simulink model "detumbling"  (R2020b)
settings: Solver=ode15s  StartTime=0  StopTime=900  MaxStep=0.1  RelTol=1e-8  AbsTol=1e-8
values from neighbouring files (symbols this model uses):
  data = struct()    [config.m]
libraries: simulink x3
settings Model: Creator=pacif  LastModifiedBy=pacif

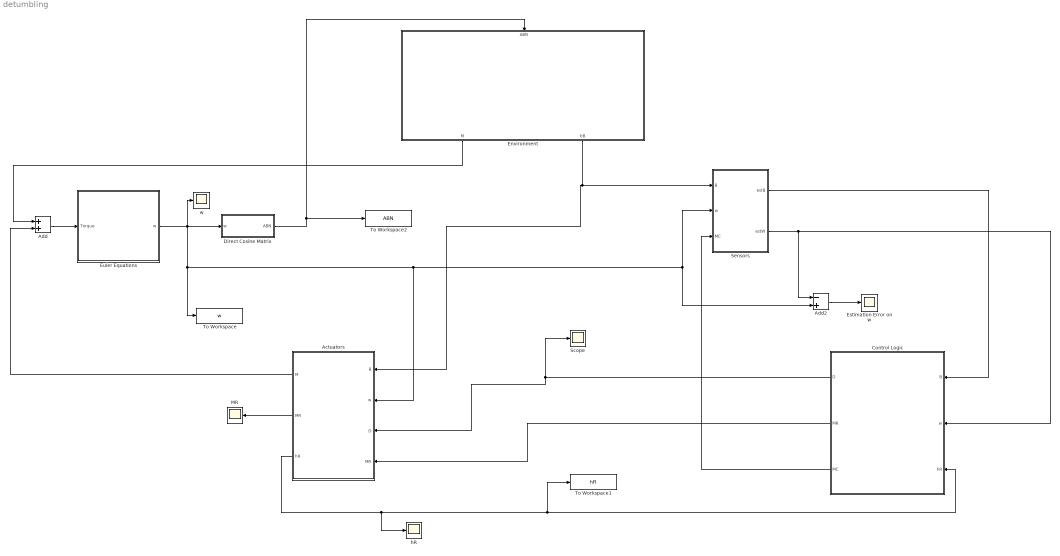
== system detumbling ==
  Actuators : Subsystem  AncestorBlock=libraryMatlab/Actuators
  Add : Sum
  Add2 : Sum  Inputs=-+
  Control Logic : Subsystem  AncestorBlock=libraryMatlab/Control Logic
  Direct Cosine Matrix : Subsystem  AncestorBlock=libraryMatlab/Direct Cosine Matrix
  Environment : Subsystem  AncestorBlock=libraryMatlab/Environment
  Estimation Error on w : Scope
  Euler Equations : Subsystem  AncestorBlock=libraryMatlab/Euler Equations
  MR : Scope
  Scope : Scope
  Sensors : Subsystem  AncestorBlock=libraryMatlab/Sensors Old
  To Workspace : ToWorkspace  VariableName=w  SaveFormat=Timeseries  SampleTime=-1
  To Workspace1 : ToWorkspace  VariableName=hR  SaveFormat=Timeseries  SampleTime=-1
  To Workspace2 : ToWorkspace  VariableName=ABN  SaveFormat=Timeseries  SampleTime=-1
  hR : Scope
  w : Scope
  wires:
  Direct Cosine Matrix/1(ABN) -> To Workspace2/1, Environment/1(ABN)
  Environment/2(bB) -> Actuators/1(B), Sensors/1(B)
  Control Logic/1(D) -> Scope/1, Actuators/3(D)
  Control Logic/2(MR) -> Actuators/4("MR ")
  Actuators/3(hR) -> hR/1, To Workspace1/1, Control Logic/3(hR)
  Sensors/2(estW) -> Add2/1, Control Logic/2(w)
  Add/1 -> Euler Equations/1(Torque)
  Actuators/1(M) -> Add/2
  Environment/1(M) -> Add/1
  Actuators/2(MR) -> MR/1
  Euler Equations/1(w) -> Actuators/2(w), Sensors/2(w), Add2/2, To Workspace/1, w/1, Direct Cosine Matrix/1(w)
  Add2/1 -> Estimation Error on w/1
  Control Logic/3(MC) -> Sensors/3(MC)
  Sensors/1(estB) -> Control Logic/1(B)

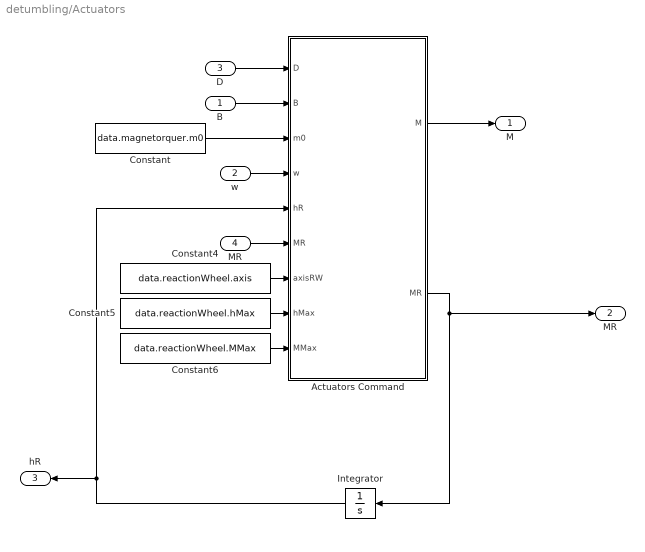
== system detumbling/Actuators ==
  B : Inport
  w : Inport  Port=2
  D : Inport  Port=3
  "MR " : Inport  Port=4
  Actuators Command : MATLAB Function  TreatAsAtomicUnit=on
  Constant : Constant  Value=data.magnetorquer.m0
  Constant4 : Constant  Value=data.reactionWheel.axis
  Constant5 : Constant  Value=data.reactionWheel.hMax
  Constant6 : Constant  Value=data.reactionWheel.MMax
  Integrator : Integrator  InitialCondition=data.reactionWheel.h0
  M : Outport
  MR : Outport  Port=2
  hR : Outport  Port=3
  wires:
  w/1 -> Actuators Command/4(w)
  Integrator/1 -> Actuators Command/5(hR), hR/1
  Actuators Command/2(MR) -> MR/1, Integrator/1
  Constant6/1 -> Actuators Command/9(MMax)
  Constant5/1 -> Actuators Command/8(hMax)
  Constant4/1 -> Actuators Command/7(axisRW)
  "MR "/1 -> Actuators Command/6("MR ")
  Actuators Command/1(M) -> M/1
  B/1 -> Actuators Command/2(B)
  D/1 -> Actuators Command/1(D)
  Constant/1 -> Actuators Command/3(m0)

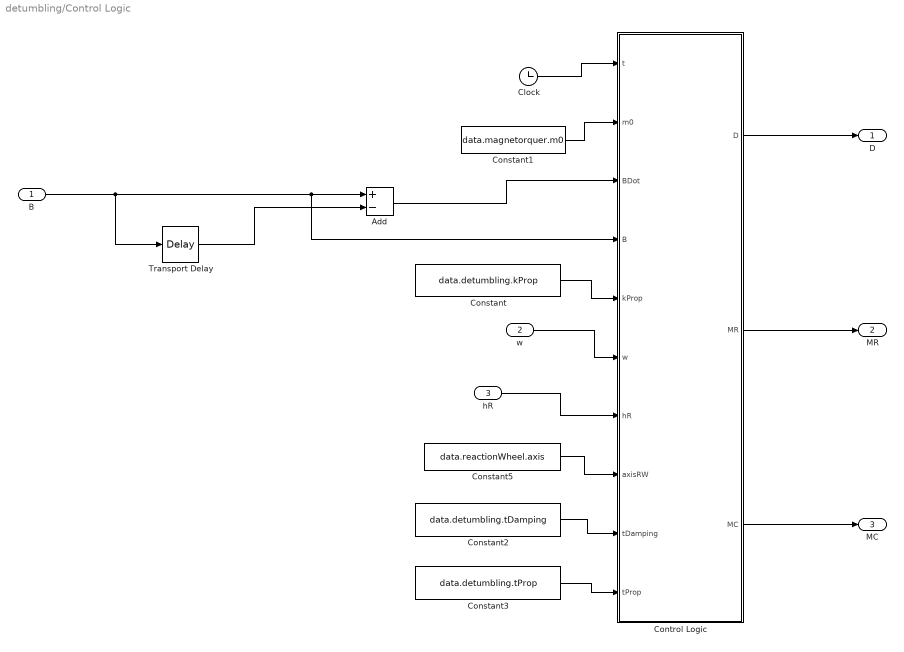
== system detumbling/Control Logic ==
  B : Inport
  w : Inport  Port=2
  hR : Inport  Port=3
  Add : Sum  Inputs=+-
  Clock : Clock
  Constant : Constant  Value=data.detumbling.kProp
  Constant1 : Constant  Value=data.magnetorquer.m0  VectorParams1D=off
  Constant2 : Constant  Value=data.detumbling.tDamping
  Constant3 : Constant  Value=data.detumbling.tProp
  Constant5 : Constant  Value=data.reactionWheel.axis
  Control Logic : MATLAB Function  TreatAsAtomicUnit=on
  Transport Delay : TransportDelay  DelayTime=data.magnetometer.sampleTime  InitialOutput=[0;0;0]
  D : Outport
  MR : Outport  Port=2
  MC : Outport  Port=3
  wires:
  Transport Delay/1 -> Add/2
  Add/1 -> Control Logic/3(BDot)
  B/1 -> Control Logic/4(B), Add/1, Transport Delay/1
  hR/1 -> Control Logic/7(hR)
  Control Logic/2(MR) -> MR/1
  Control Logic/1(D) -> D/1
  Constant5/1 -> Control Logic/8(axisRW)
  w/1 -> Control Logic/6(w)
  Constant1/1 -> Control Logic/2(m0)
  Constant/1 -> Control Logic/5(kProp)
  Clock/1 -> Control Logic/1(t)
  Constant2/1 -> Control Logic/9(tDamping)
  Constant3/1 -> Control Logic/10(tProp)
  Control Logic/3(MC) -> MC/1

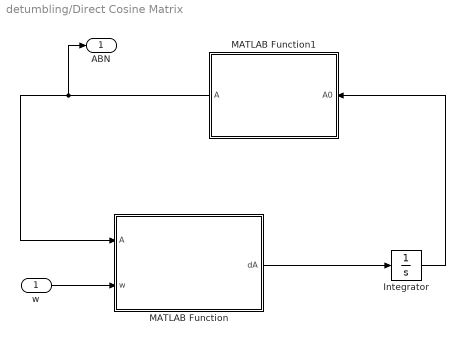
== system detumbling/Direct Cosine Matrix ==
  w : Inport
  Integrator : Integrator  InitialCondition=data.ic.dcm
  MATLAB Function : MATLAB Function  TreatAsAtomicUnit=on
  MATLAB Function1 : MATLAB Function  TreatAsAtomicUnit=on
  ABN : Outport
  wires:
  MATLAB Function1/1(A) -> MATLAB Function/1(A), ABN/1
  Integrator/1 -> MATLAB Function1/1(A0)
  MATLAB Function/1(dA) -> Integrator/1
  w/1 -> MATLAB Function/2(w)

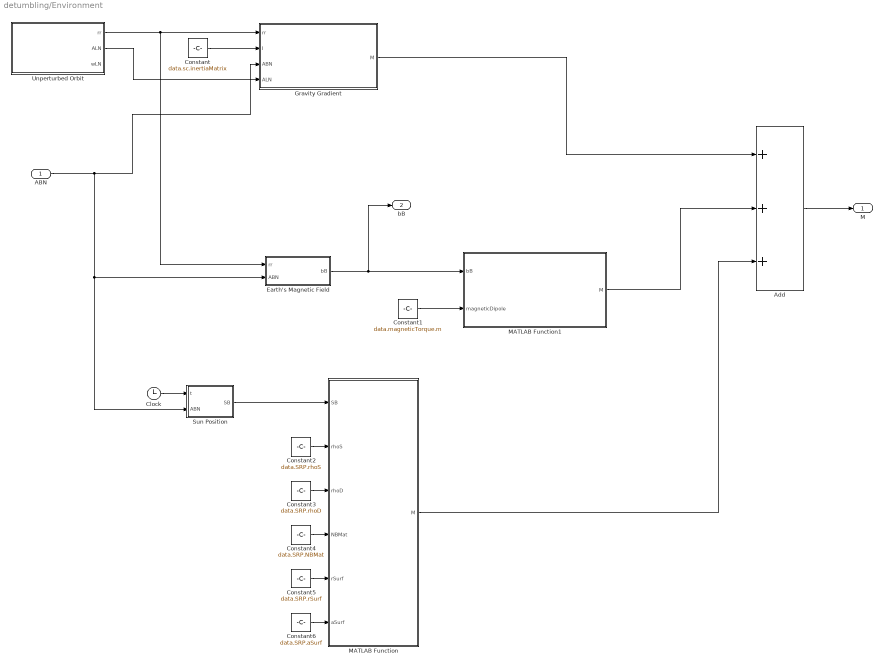
== system detumbling/Environment ==
  ABN : Inport
  Add : Sum  Inputs=+++
  Clock : Clock
  Constant : Constant  Value=data.sc.inertiaMatrix
  Constant1 : Constant  Value=data.magneticTorque.m
  Constant2 : Constant  Value=data.SRP.rhoS
  Constant3 : Constant  Value=data.SRP.rhoD
  Constant4 : Constant  Value=data.SRP.NBMat
  Constant5 : Constant  Value=data.SRP.rSurf
  Constant6 : Constant  Value=data.SRP.aSurf
  Earth's Magnetic Field : Subsystem
  Gravity Gradient : MATLAB Function  TreatAsAtomicUnit=on
  MATLAB Function : MATLAB Function  TreatAsAtomicUnit=on
  MATLAB Function1 : MATLAB Function  TreatAsAtomicUnit=on
  Sun Position : MATLAB Function  TreatAsAtomicUnit=on
  Unperturbed Orbit : Subsystem
  M : Outport
  bB : Outport  Port=2
  wires:
  Sun Position/1(SB) -> MATLAB Function/1(SB)
  Clock/1 -> Sun Position/1(t)
  Constant4/1 -> MATLAB Function/4(NBMat)
  Constant6/1 -> MATLAB Function/6(aSurf)
  Constant3/1 -> MATLAB Function/3(rhoD)
  Constant2/1 -> MATLAB Function/2(rhoS)
  Constant5/1 -> MATLAB Function/5(rSurf)
  ABN/1 -> Earth's Magnetic Field/2(ABN), Sun Position/2(ABN), Gravity Gradient/3(ABN)
  Add/1 -> M/1
  MATLAB Function/1(M) -> Add/3
  Gravity Gradient/1(M) -> Add/1
  Earth's Magnetic Field/1(bB) -> MATLAB Function1/1(bB), bB/1
  MATLAB Function1/1(M) -> Add/2
  Constant1/1 -> MATLAB Function1/2(magneticDipole)
  Constant/1 -> Gravity Gradient/2(I)
  Unperturbed Orbit/2(ALN) -> Gravity Gradient/4(ALN)
  Unperturbed Orbit/1(rr) -> Gravity Gradient/1(rr), Earth's Magnetic Field/1(rr)

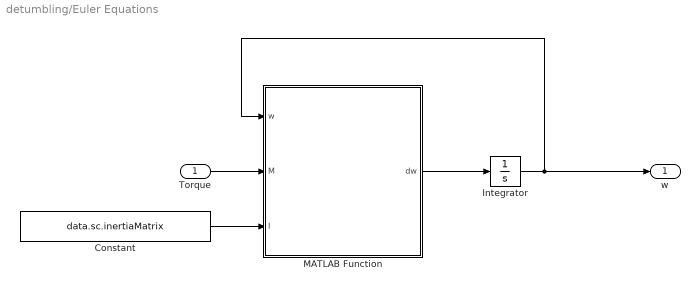
== system detumbling/Euler Equations ==
  Torque : Inport
  Constant : Constant  Value=data.sc.inertiaMatrix
  Integrator : Integrator  InitialCondition=data.ic.w
  MATLAB Function : MATLAB Function  TreatAsAtomicUnit=on
  w : Outport
  wires:
  MATLAB Function/1(dw) -> Integrator/1
  Torque/1 -> MATLAB Function/2(M)
  Integrator/1 -> MATLAB Function/1(w), w/1
  Constant/1 -> MATLAB Function/3(I)

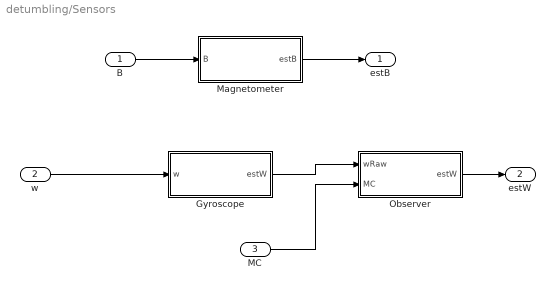
== system detumbling/Sensors ==
  B : Inport
  w : Inport  Port=2
  MC : Inport  Port=3
  Gyroscope : Subsystem
  Magnetometer : Subsystem
  Observer : Subsystem
  estB : Outport
  estW : Outport  Port=2
  wires:
  Magnetometer/1(estB) -> estB/1
  B/1 -> Magnetometer/1(B)
  Observer/1(estW) -> estW/1
  w/1 -> Gyroscope/1(w)
  Gyroscope/1(estW) -> Observer/1(wRaw)
  MC/1 -> Observer/2(MC)

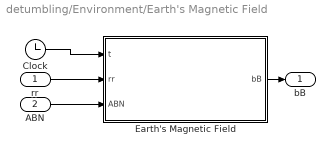
== system detumbling/Environment/Earth's Magnetic Field ==
  rr : Inport
  ABN : Inport  Port=2
  Clock : Clock
  Earth's Magnetic Field : MATLAB Function  TreatAsAtomicUnit=on
  bB : Outport
  wires:
  Clock/1 -> Earth's Magnetic Field/1(t)
  ABN/1 -> Earth's Magnetic Field/3(ABN)
  rr/1 -> Earth's Magnetic Field/2(rr)
  Earth's Magnetic Field/1(bB) -> bB/1

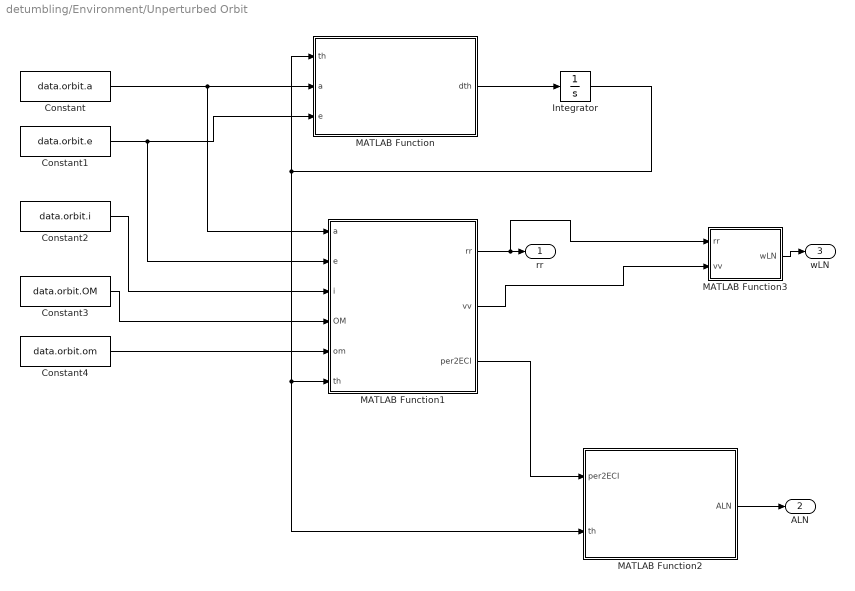
== system detumbling/Environment/Unperturbed Orbit ==
  Constant : Constant  Value=data.orbit.a
  Constant1 : Constant  Value=data.orbit.e
  Constant2 : Constant  Value=data.orbit.i
  Constant3 : Constant  Value=data.orbit.OM
  Constant4 : Constant  Value=data.orbit.om
  Integrator : Integrator  InitialCondition=data.ic.th
  MATLAB Function : MATLAB Function  TreatAsAtomicUnit=on
  MATLAB Function1 : MATLAB Function  TreatAsAtomicUnit=on
  MATLAB Function2 : MATLAB Function  TreatAsAtomicUnit=on
  MATLAB Function3 : MATLAB Function  TreatAsAtomicUnit=on
  rr : Outport
  ALN : Outport  Port=2
  wLN : Outport  Port=3
  wires:
  MATLAB Function3/1(wLN) -> wLN/1
  MATLAB Function2/1(ALN) -> ALN/1
  MATLAB Function1/3(per2ECI) -> MATLAB Function2/1(per2ECI)
  MATLAB Function1/2(vv) -> MATLAB Function3/2(vv)
  MATLAB Function1/1(rr) -> rr/1, MATLAB Function3/1(rr)
  Constant4/1 -> MATLAB Function1/5(om)
  Constant3/1 -> MATLAB Function1/4(OM)
  Constant2/1 -> MATLAB Function1/3(i)
  Integrator/1 -> MATLAB Function/1(th), MATLAB Function1/6(th), MATLAB Function2/2(th)
  MATLAB Function/1(dth) -> Integrator/1
  Constant1/1 -> MATLAB Function/3(e), MATLAB Function1/2(e)
  Constant/1 -> MATLAB Function/2(a), MATLAB Function1/1(a)

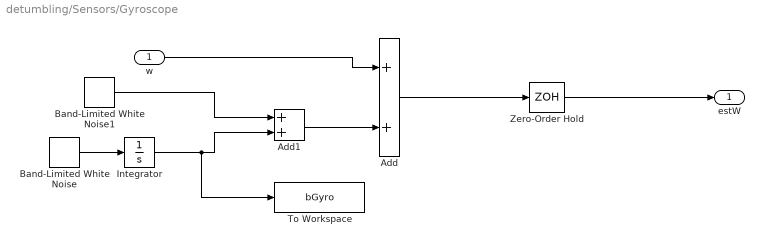
== system detumbling/Sensors/Gyroscope ==
  w : Inport
  Add : Sum
  Add1 : Sum
  Band-Limited White Noise : simulink/Sources/Band-Limited White Noise  Cov=data.gyroscope.sigmaB^2*[1;1;1]  Ts=data.gyroscope.sampleTime  seed=[0;1;2]
  Band-Limited White Noise1 : simulink/Sources/Band-Limited White Noise  Cov=data.gyroscope.sigmaN^2*[1;1;1]  Ts=data.gyroscope.sampleTime  seed=[43;332;234]
  Integrator : Integrator  InitialCondition=data.gyroscope.b0
  To Workspace : ToWorkspace  VariableName=bGyro  SaveFormat=Timeseries  SampleTime=-1
  Zero-Order Hold : ZeroOrderHold  SampleTime=data.gyroscope.sampleTime
  estW : Outport
  wires:
  Zero-Order Hold/1 -> estW/1
  Add/1 -> Zero-Order Hold/1
  Band-Limited White Noise1/1 -> Add1/1
  Integrator/1 -> To Workspace/1, Add1/2
  Add1/1 -> Add/2
  w/1 -> Add/1
  Band-Limited White Noise/1 -> Integrator/1

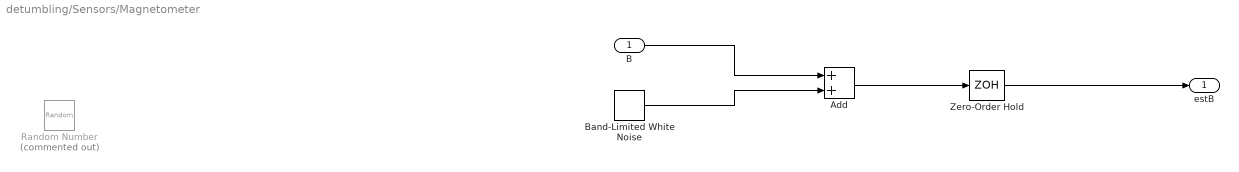
== system detumbling/Sensors/Magnetometer ==
  B : Inport
  Add : Sum
  Band-Limited White Noise : simulink/Sources/Band-Limited White Noise  Cov=(data.magnetometer.sigma)^2*[1;1;1]  Ts=data.magnetometer.sampleTime  seed=[23341;232434;232124]
  Random Number : RandomNumber  Commented=on  Mean=[0;0;0]  Variance=(data.magnetometer.sigma)^2*[1;1;1]  SampleTime=data.magnetometer.sampleTime
  Zero-Order Hold : ZeroOrderHold  SampleTime=data.magnetometer.sampleTime
  estB : Outport
  wires:
  Band-Limited White Noise/1 -> Add/2
  Add/1 -> Zero-Order Hold/1
  Zero-Order Hold/1 -> estB/1
  B/1 -> Add/1

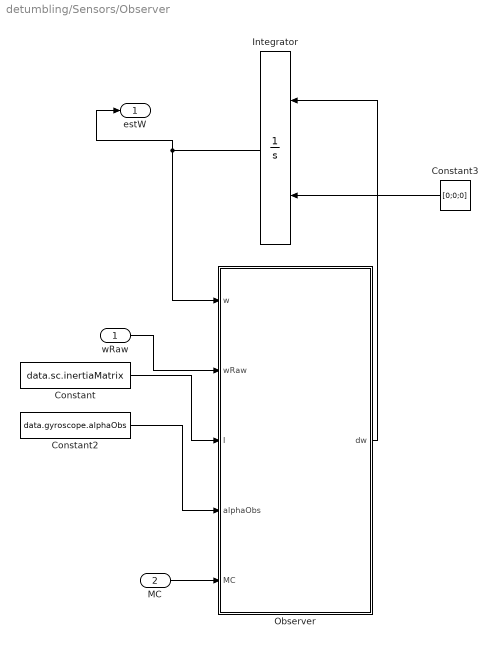
== system detumbling/Sensors/Observer ==
  wRaw : Inport
  MC : Inport  Port=2
  Constant : Constant  Value=data.sc.inertiaMatrix
  Constant2 : Constant  Value=data.gyroscope.alphaObs
  Constant3 : Constant  Value=[0;0;0]
  Integrator : Integrator  InitialConditionSource=external
  Observer : MATLAB Function  TreatAsAtomicUnit=on
  estW : Outport
  wires:
  wRaw/1 -> Observer/2(wRaw)
  Constant/1 -> Observer/3(I)
  Observer/1(dw) -> Integrator/1
  Integrator/1 -> estW/1, Observer/1(w)
  Constant2/1 -> Observer/4(alphaObs)
  MC/1 -> Observer/5(MC)
  Constant3/1 -> Integrator/2

== matlab function detumbling/Environment/MATLAB Function1 ==
  data: bB input; M output; magneticDipole input
function M = magneticTorque(bB,magneticDipole)

M = cross(magneticDipole,bB); 

end

== matlab function detumbling/Environment/MATLAB Function ==
  data: SB input; rhoS input; rhoD input; NBMat input; rSurf input; aSurf input; M output
function M = SRP(SB,rhoS,rhoD,NBMat,rSurf,aSurf)

% Constants:
Fe = 2081.4; c = 3e8; P = Fe/c;

nSurf = size(NBMat,2);

M = [0; 0; 0];

for i = 1:nSurf
    
    NBi = NBMat(:,i); ri = rSurf(:,i); Ai = aSurf(i);
    rhoSi = rhoS(i); rhoDi = rhoD(i);
    
    Ki = dot(SB,NBi); 
    
    if Ki > 0
        
        Fi = -P*Ai*Ki*((1-rhoSi)*SB +...
            (2*rhoSi*Ki + 2/3*rhoDi)*NBi);
        
        M = M + cross(ri,Fi);
        
    end
    
end

end

== matlab function detumbling/Environment/Earth's Magnetic Field/Earth's Magnetic Field ==
  data: t input; bB output; rr input; ABN input
function bB = fcn(t,rr,ABN)

% Coefficients for 2020:
g10 = -29615e-9; g11 = -1728e-9; h11 = 5186e-9;
H0 = sqrt(g10^2 + g11^2 + h11^2);

OBL = 11.5*pi/180;
W_EARTH = (2*pi + 2*pi/365.26)/24/3600;
R_EARTH = 6371.0088;

mVers = [sin(OBL)*cos(W_EARTH*t);
        sin(OBL)*sin(W_EARTH*t);
        cos(OBL)];

rVers = rr/norm(rr);
rNorm = norm(rr);

bN = R_EARTH^3/rNorm^3*H0*(3*dot(mVers,rVers)*rVers - mVers);

bB = ABN*bN;

end

== matlab function detumbling/Environment/Unperturbed Orbit/MATLAB Function3 ==
  data: rr input; wLN output; vv input
function wLN = fcn(rr,vv)

MU = 398600;

n = sqrt(MU/(norm(rr)^3));

h = cross(rr,vv); 

wLN = h/norm(h)*n;

== matlab function detumbling/Environment/Sun Position ==
  data: t input; SB output; ABN input
function SB = fcn(t,ABN)

N_SUN = 2*pi/365/24/3600; OBL = 23.45*pi/180;
R_SUN = 1.496e8;

SN = R_SUN*[cos(N_SUN*t); 
    sin(N_SUN*t)*cos(OBL);
    sin(N_SUN*t)*sin(OBL)];
SN = SN/norm(SN);

SB = ABN*SN;

== matlab function detumbling/Actuators/Actuators Command ==
  data: D input; M output; MR output; B input; m0 input; w input; hR input; MR input; axisRW input; hMax input; MMax input
function [M,MR] = fcn(D, B, m0, w, hR, MR, axisRW, hMax, MMax)

% Magnetorquers:
for i = 1:3
    D(i) = min(D(i),m0); D(i) = max(D(i),-m0);
end
MMagn = cross(D,B);

% Reaction Wheels:
for i = 1:length(MR)
    
    if abs(MR(i)) > MMax; MR(i) = sign(MR(i))*MMax; end
    if hR(i) >= hMax && MR(i) > 0, MR(i) = 0; end
    if hR(i) <= -hMax && MR(i) < 0, MR(i) = 0; end
    
end

MRW = -cross(w,axisRW*hR) - axisRW*MR;

M = MMagn + MRW;

== matlab function detumbling/Control Logic/Control Logic ==
  data: D output; MR output; MC output; t input; m0 input; BDot input; B input; kProp input; w input; hR input; axisRW input; tDamping input; tProp input
function [D,MR,MC] = fcn(t,m0,BDot,B,kProp,w,hR,axisRW,tDamping,tProp)

D = [0;0;0]; MR = 0*axisRW(1,:)'; MC = [0;0;0];

if t > 0 && t < tDamping
    
    D = -m0*sign(BDot);
    
    MC = cross(D,B);

elseif t > tDamping && t < tProp
    
    MC = - kProp*w;
    
    MC1 = MC + cross(w,axisRW*hR);
    
    D = cross(B,MC1)/norm(B)^2;
    
    for i = 1:3
        D(i) = min(D(i),m0); D(i) = max(D(i),-m0);
    end
    
    MEff = cross(D,B);
    
    MC2 = MC1 - MEff;
    
    MR = -pinv(axisRW)*(MC2 + cross(w,axisRW*hR));
    
end

== matlab function detumbling/Direct Cosine Matrix/MATLAB Function ==
  data: A input; dA output; w input
function dA = derivativeDCM(A,w)

M = [ 0 -w(3) w(2); 
    w(3) 0 -w(1);
    -w(2) w(1) 0];

dA = -M*A;


end

== matlab function detumbling/Euler Equations/MATLAB Function ==
  data: w input; dw output; M input; I input
function dw = eulerEquations(w,M,I)

dw = I\(cross(I*w,w) + M);

end

== matlab function detumbling/Direct Cosine Matrix/MATLAB Function1 ==
  data: A0 input; A output
function A = orthonormalizeA(A0)

A = A0*3/2 - A0*(A0')*A0/2;

end

== matlab function detumbling/Sensors/Observer/Observer ==
  data: w input; dw output; wRaw input; I input; alphaObs input; MC input
function dw = fcn(w,wRaw,I,alphaObs,MC)

dw = I\cross(I*w,w) + I\MC - alphaObs*(w - wRaw);

== matlab function detumbling/Environment/Gravity Gradient ==
  data: rr input; M output; I input; ABN input; ALN input
function M = fun(rr,I,ABN,ALN)

MU = 398600;

Ix = I(1,1); Iy = I(2,2); Iz = I(3,3);

R = norm(rr);

ABL = ABN*ALN';

c = ABL*[1;0;0];

K = 3*MU/R^3;

M = K*[ (Iz - Iy)*c(3)*c(2);
        (Ix - Iz)*c(1)*c(3);
        (Iy - Ix)*c(2)*c(1)  ];
    
end

== matlab function detumbling/Environment/Unperturbed Orbit/MATLAB Function ==
  data: th input; dth output; a input; e input
function dth = thetaDot(th, a, e)

MU = 398600;

n = sqrt(MU/a^3);

dth = n*(1 + e*cos(th))^2/(1 - e^2)^(3/2);

end

== matlab function detumbling/Environment/Unperturbed Orbit/MATLAB Function1 ==
  data: a input; rr output; e input; i input; OM input; om input; th input; vv output; per2ECI output
function [rr,vv,per2ECI] = kep2car(a,e,i,OM,om,th)

MU = 398600;

p = a*(1-e^2);
r = p/(1+e*cos(th));

rr = r*[cos(th);sin(th);0];
vv = sqrt(MU/p)*[-sin(th);e+cos(th);0];

ROM = [ cos(OM) sin(OM) 0; -sin(OM) cos(OM) 0; 0 0 1];
Ri = [ 1 0 0; 0 cos(i) sin(i); 0 -sin(i) cos(i)];
Rom = [ cos(om) sin(om) 0; -sin(om) cos(om) 0; 0 0 1];

per2ECI = (Rom*Ri*ROM)';

rr = per2ECI*rr;
vv = per2ECI*vv;

end

== matlab function detumbling/Environment/Unperturbed Orbit/MATLAB Function2 ==
  data: per2ECI input; ALN output; th input
function ALN = computeALN(per2ECI,th)

ECI2per = per2ECI';

per2L = [cos(th)  sin(th)  0;
        -sin(th)  cos(th)  0;
            0        0     1];
        
ALN = per2L*ECI2per;

end
